simulink model "lincobelli_mdl"  (Simulink 7.8)
settings: Solver=ode4  StartTime=0.0  StopTime=t_span  RelTol=1e-3
values from neighbouring files (symbols this model uses):
  par = cobelli_start(:,icount)    [cobelli_error_generate.m]    (also in generate_target_free_cobelli.m = [k21,k12,Vm,Km,k02,c1,b1,V1,VE]; generate_target_impulse_cobelli.m = [k21,k12,Vm,Km,k02,c1,b1,V1,VE]; generate_target_step_cobelli.m = [k21,k12,Vm,Km,k02,c1,b1,V1,VE]; test_cobelli_error.m = [k21,k12,Vm,Km,k02,c1,b1,V1,VE])
  x_i = 0    [cobelli_error.m]    (also in cobelli_error_mdl.m; free_cobelli.m = 0.2; generate_target_free_cobelli.m = 0.2; generate_target_impulse_cobelli.m)
undefined symbols (not defined in the file or in its folder): outstr1, params
settings Model: Creator=Kourosh Danai  LastModifiedBy=BionicBill
settings DataIOCC: SaveFormat=StructureWithTime  TimeSaveName=t  OutputSaveName=y
settings DebuggingCC: AlgebraicLoopMsg=none  FcnCallInpInsideContextMsg=Use local settings  StrictBusMsg=Warning
settings SFSimCC: SimParseCustomCode=off

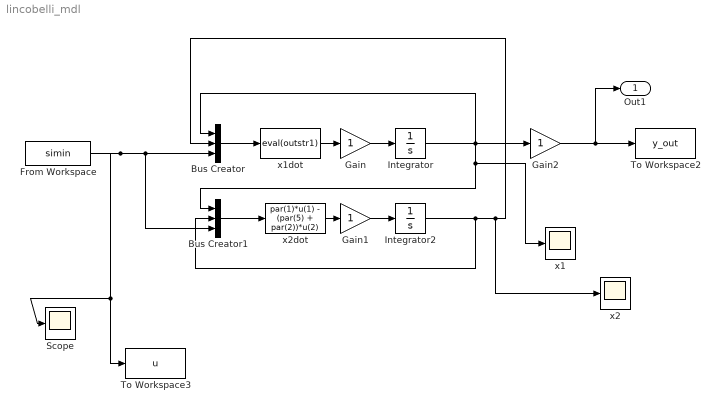
== system lincobelli_mdl ==
  Bus Creator : BusCreator  Inputs=3
  Bus Creator1 : BusCreator  Inputs=3
  From Workspace : FromWorkspace  VariableName=simin  SampleTime=params.simulation.samp_time
  Gain : Gain
  Gain1 : Gain
  Gain2 : Gain
  Integrator : Integrator  InitialCondition=x_i
  Integrator2 : Integrator
  Scope : Scope
  To Workspace2 : ToWorkspace  VariableName=y_out  SampleTime=-1  SaveFormat=Array
  To Workspace3 : ToWorkspace  VariableName=u  SampleTime=-1  SaveFormat=Array
  x1 : Scope
  x1dot : MATLABFcn  MATLABFcn=eval(outstr1)
  x2 : Scope
      settings: SaveName=ScopeData2
  x2dot : MATLABFcn  MATLABFcn=par(1)*u(1) - (par(5) + par(2))*u(2)
  Out1 : Outport
  wires:
  Bus Creator/1 -> x1dot/1
  Gain/1 -> Integrator/1
  x1dot/1 -> Gain/1
  Bus Creator1/1 -> x2dot/1
  Gain1/1 -> Integrator2/1
  x2dot/1 -> Gain1/1
  Integrator/1 -> Bus Creator/1, Bus Creator1/1, x1/1, Gain2/1
  Integrator2/1 -> Bus Creator1/2, Bus Creator/2, x2/1
  Gain2/1 -> To Workspace2/1, Out1/1
  From Workspace/1 -> Bus Creator/3, Bus Creator1/3, To Workspace3/1, Scope/1
